simulink model "Bien1_simu"  (Simulink 9.1)
settings: Solver=VariableStepAuto  StartTime=0.0  StopTime=10.0  RelTol=1e-3
values from neighbouring files (symbols this model uses):
  m = [(m1*lc1^2)+m2*(l1^2+lc2^2+2*l1*lc2*cos(q2))+I1+I2 (m2*(lc2^2+l1*lc2*m2*cos(q2)+I2)) ... (first row only)    [brazomire.m]    (also in examvib3.m = 0.2533; fft estatica.m = [0:0.02:100]; fftestatica.m = [0:0.02:100])
  N = cat(1,N,b)    [ackerobs.m]    (also in espectograma.m = 128)
undefined symbols (not defined in the file or in its folder): As, Bs, CC, KK, uq, xq
libraries: mblibv1 x17
settings Model: LogicAnalyzerSignalOrdering=b2078105-ca7e-427e-be0d-a23da488db86  Creator=Dell  LastModifiedBy=Dell
settings DataIOCC: SaveFormat=Dataset
settings OptimizationCC: LifeSpan=auto
settings DebuggingCC: UnderspecifiedInitializationDetection=Simplified  MergeDetectMultiDrivingBlocksExec=error  SFUnexpectedBacktrackingDiag=error  SFNoUnconditionalDefaultTransitionDiag=error  SFExecutionAtInitializationDiag=warning
settings HardwareCC: ProdBitPerPointer=64  ProdBitPerSizeT=64  ProdBitPerPtrDiffT=64  ProdLargestAtomicFloat=Float  ProdIntDivRoundTo=Zero  ProdEndianess=LittleEndian  ProdWordSize=64  ProdHWDeviceType=Intel->x86-64 (Windows64)
settings ModelReferenceCC: PropagateSignalLabelsOutOfModel=on
settings GRTTargetCC: TargetLangStandard=C99 (ISO)  CombineOutputUpdateFcns=on  GRTInterface=off
settings ConfigComp: CovMetricSettings=dwe  CovHtmlReporting=off  CovSaveCumulativeToWorkspaceVar=off  CovSaveSingleToWorkspaceVar=off  CovExternalEMLEnable=on
settings SimscapeCC: SimscapeNormalizeSystem=off

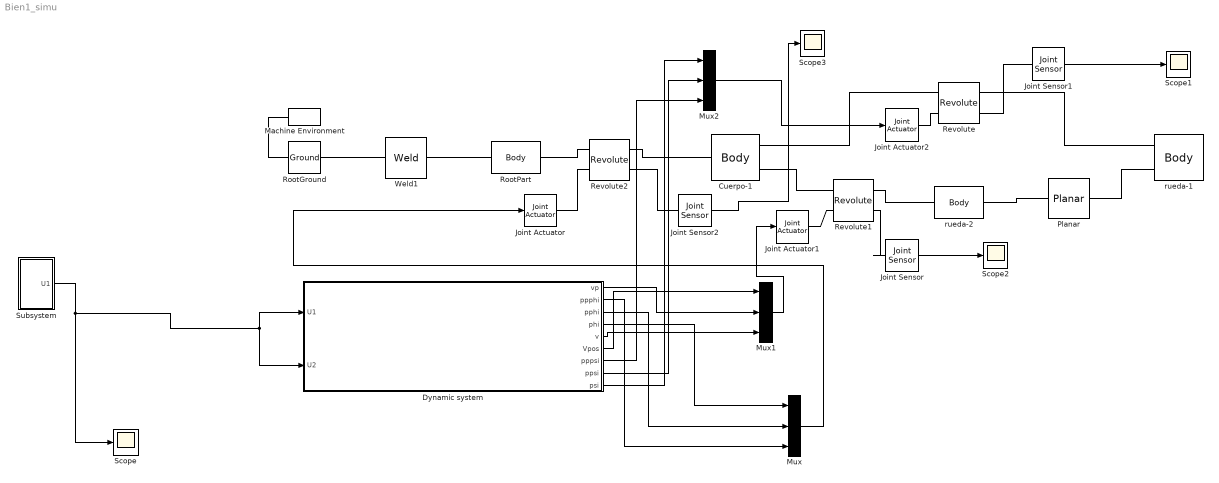
== system Bien1_simu ==
  Cuerpo-1 : mblibv1/Bodies/Body  LConnTagsString=CS2  RConnTagsString=CS3|CS4  UpdateFromCAD=on  DialogClass=MechanicalBodyBlock  Mass=0.199965  MassUnits=kg  InertiaUnits=kg*m^2  Inertia=[0.00141468,0,-1.2536e-08;0,0.00138764,6.39875e-09;-1.2536e-08,6.39875e-09,0.0027923]  Shape=Cylinder  ShapeDims=[1 1]  ShapeUnits=m  ShapeUse=false  Density=1  DensityUnits=kg/m^3  DensityUse=false  GraphicsMode=GFXFILE  GraphicsFileName=Segway - Cuerpo-1.STL  BodyColorSelMode=COLORPALETTE  BodyColor=[0.647059;0.619608;0.588235]  AttachedToCS=CS1  CG=Right$CG$[0.00341994 -0.0544159 8.19624e-07]$WORLD$WORLD$m$[1 0 0;0 1 0;0 0 1]$3x3 Transform$rad$WORLD$false$none  WorkingFrames=Right$CS1$[-0.18408 -0.111622 0]$WORLD$WORLD$m$[1 0 0;0 1 0;0 0 1]$3x3 Transform$rad$WORLD$false$none#Left$CS2$[0.00341994 -0.0544159 8.19624e-07]$WORLD$WORLD$m$[1 0 0;0 1 0;0 0 1]$3x3 Transform$rad$WORLD$true$none#Right$CS3$[0.19092 -0.111622 0]$WORLD$WORLD$m$[1 0 0;0 1 0;0 0 1]$3x3 Transform$rad$WORLD$true$none#Right$CS4$[0.19092 -0.111622 0]$WORLD$WORLD$m$[1 0 0;0 1 0;0 0 1]$3x3 Transform$rad$WORLD$true$none  CGPos=[0.00341994 -0.0544159 8.19624e-07]  CGRot=[1 0 0;0 1 0;0 0 1]  CS0Pos=[]  CS0Rot=[]  CS1Pos=[-0.18408 -0.111622 0]  CS1Rot=[1 0 0;0 1 0;0 0 1]  CS2Pos=[0.00341994 -0.0544159 8.19624e-07]  CS2Rot=[1 0 0;0 1 0;0 0 1]  CS3Pos=[0.19092 -0.111622 0]  CS3Rot=[1 0 0;0 1 0;0 0 1]  CS4Pos=[0.19092 -0.111622 0]  CS4Rot=[1 0 0;0 1 0;0 0 1]  CS5Pos=[]  CS5Rot=[]  CS6Pos=[]  CS6Rot=[]  CS7Pos=[]  CS7Rot=[]  CS8Pos=[]  CS8Rot=[]  CS9Pos=[]  CS9Rot=[]  CS10Pos=[]  CS10Rot=[]  CS11Pos=[]  CS11Rot=[]  CS12Pos=[]  CS12Rot=[]  CS13Pos=[]  CS13Rot=[]  CS14Pos=[]  CS14Rot=[]  CS15Pos=[]  CS15Rot=[]  CS16Pos=[]  CS16Rot=[]  CS17Pos=[]  CS17Rot=[]  CS18Pos=[]  CS18Rot=[]  CS19Pos=[]  CS19Rot=[]  CS20Pos=[]  CS20Rot=[]
      settings: SourceProductName=Simscape Multibody  SourceProductBaseCode=MS
  Dynamic system : Subsystem
  Joint Actuator : mblibv1/Sensors &  Actuators/Joint Actuator  UpdateFromCAD=off  PhysicalDomain=Mechanical  PortType=blob  ActuationStyle=Motion  AngleUnits=deg  ArcVelocityUnits=deg/s  ArcAccelerationUnits=deg/s^2  CoordPositionUnits=m  VelocityUnits=m/s  AccelerationUnits=m/s^2  ForceUnits=N  TorqueUnits=N*m  ActiveIO=on  Width=3  DialogClass=MechanicalActuatorBlock  Primitive=R1  ReferenceFrame=Absolute (World)
      settings: SourceProductName=Simscape Multibody  SourceProductBaseCode=MS
  Joint Actuator1 : mblibv1/Sensors &  Actuators/Joint Actuator  UpdateFromCAD=off  PhysicalDomain=Mechanical  PortType=blob  ActuationStyle=Motion  AngleUnits=deg  ArcVelocityUnits=rad/s  ArcAccelerationUnits=deg/s^2  CoordPositionUnits=m  VelocityUnits=m/s  AccelerationUnits=m/s^2  ForceUnits=N  TorqueUnits=N*m  ActiveIO=on  Width=3  DialogClass=MechanicalActuatorBlock  Primitive=R1  ReferenceFrame=Absolute (World)
      settings: SourceProductName=Simscape Multibody  SourceProductBaseCode=MS
  Joint Actuator2 : mblibv1/Sensors &  Actuators/Joint Actuator  UpdateFromCAD=off  PhysicalDomain=Mechanical  PortType=blob  ActuationStyle=Motion  AngleUnits=deg  ArcVelocityUnits=deg/s  ArcAccelerationUnits=deg/s^2  CoordPositionUnits=m  VelocityUnits=m/s  AccelerationUnits=m/s^2  ForceUnits=N  TorqueUnits=N*m  ActiveIO=on  Width=3  DialogClass=MechanicalActuatorBlock  Primitive=R1  ReferenceFrame=Absolute (World)
      settings: SourceProductName=Simscape Multibody  SourceProductBaseCode=MS
  Joint Sensor : mblibv1/Sensors &  Actuators/Joint Sensor  UpdateFromCAD=off  PhysicalDomain=Mechanical  PortType=blob  Muxed=on  Pose=off  Angle=on  AngleUnits=deg  ArcVelocity=off  ArcVelocityUnits=deg/s  ArcAcceleration=off  ArcAccelerationUnits=deg/s^2  CoordPosition=on  CoordPositionUnits=m  Velocity=off  VelocityUnits=m/s  Acceleration=off  AccelerationUnits=m/s^2  Quaternion=on  QuaternionDT=off  QuaternionDDT=off  QuaternionUnits=off  OutputVector=[1]  ActiveIO=on  Width=1  DialogClass=MechanicalSensorBlock  Primitive=R1  Force=off  ForceUnits=N  Torque=off  TorqueUnits=N-m  ReferenceFrame=Absolute (World)  ReactionSensedSide=Base  ReactionReferenceFrame=Absolute (World)  ReactionForce=off  ReactionForceUnits=N  ReactionMoment=off  ReactionMomentUnits=N-m
      settings: SourceProductName=Simscape Multibody  SourceProductBaseCode=MS
  Joint Sensor1 : mblibv1/Sensors &  Actuators/Joint Sensor  UpdateFromCAD=off  PhysicalDomain=Mechanical  PortType=blob  Muxed=on  Pose=off  Angle=on  AngleUnits=deg  ArcVelocity=off  ArcVelocityUnits=deg/s  ArcAcceleration=off  ArcAccelerationUnits=deg/s^2  CoordPosition=on  CoordPositionUnits=m  Velocity=off  VelocityUnits=m/s  Acceleration=off  AccelerationUnits=m/s^2  Quaternion=on  QuaternionDT=off  QuaternionDDT=off  QuaternionUnits=off  OutputVector=[1]  ActiveIO=on  Width=1  DialogClass=MechanicalSensorBlock  Primitive=R1  Force=off  ForceUnits=N  Torque=off  TorqueUnits=N-m  ReferenceFrame=Absolute (World)  ReactionSensedSide=Base  ReactionReferenceFrame=Absolute (World)  ReactionForce=off  ReactionForceUnits=N  ReactionMoment=off  ReactionMomentUnits=N-m
      settings: SourceProductName=Simscape Multibody  SourceProductBaseCode=MS
  Joint Sensor2 : mblibv1/Sensors &  Actuators/Joint Sensor  UpdateFromCAD=off  PhysicalDomain=Mechanical  PortType=blob  Muxed=on  Pose=off  Angle=on  AngleUnits=deg  ArcVelocity=off  ArcVelocityUnits=deg/s  ArcAcceleration=off  ArcAccelerationUnits=deg/s^2  CoordPosition=on  CoordPositionUnits=m  Velocity=off  VelocityUnits=m/s  Acceleration=off  AccelerationUnits=m/s^2  Quaternion=on  QuaternionDT=off  QuaternionDDT=off  QuaternionUnits=off  OutputVector=[1]  ActiveIO=on  Width=1  DialogClass=MechanicalSensorBlock  Primitive=R1  Force=off  ForceUnits=N  Torque=off  TorqueUnits=N-m  ReferenceFrame=Absolute (World)  ReactionSensedSide=Base  ReactionReferenceFrame=Absolute (World)  ReactionForce=off  ReactionForceUnits=N  ReactionMoment=off  ReactionMomentUnits=N-m
      settings: SourceProductName=Simscape Multibody  SourceProductBaseCode=MS
  Machine Environment : mblibv1/Bodies/Machine Environment  PortType=env  PhysicalDomain=Mechanical  DialogTemplateClass=MECH.MachineEnvironment  SyncWhenCopied=off  Gravity=[0 -9.81 0]  GravityUnits=m/s^2  GravityAsSignal=off  Dimensionality=Auto-detect  AnalysisType=Forward dynamics  LinearAssemblyTolerance=1e-3  LinearAssemblyToleranceUnits=m  AngularAssemblyTolerance=1e-3  AngularAssemblyToleranceUnits=rad  ConstraintSolverType=Stabilizing  ConstraintRelTolerance=1e-4  ConstraintAbsTolerance=1e-4  UseRobustSingularityHandling=off  RedundancyAnalysisToleranceType=Automatically select tolerance  RedundancyAnalysisTolerance=1e-14  StatePerturbationType=Fixed  PerturbationSize=1e-5  VisualizeMachine=on  BodyVisualizationType=Use model default body geometries  BodyColorSelMode=Use model default  DefaultBodyColor=[1 0 0]
      settings: SourceProductName=Simscape Multibody  SourceProductBaseCode=MS
  Mux : Mux  Inputs=3
  Mux1 : Mux  Inputs=3
  Mux2 : Mux  Inputs=3
  Planar : mblibv1/Joints/Planar  LConnTagsString=__newl0  RConnTagsString=__newr0  UpdateFromCAD=on  NumSAPorts=0  CutJoint=off  MarkAsCut=off  Primitives=prismatic_prismatic  PrimitiveProps=P1$WORLD$[0,1,0]$prismatic#P2$WORLD$[0,0,1]$prismatic#R1$WORLD$[-1,0,0]$revolute  DialogClass=JointBlock  P1Axis=[0,1,0]  P2Axis=[0,0,1]  R1Axis=[-1,0,0]
      settings: SourceProductName=Simscape Multibody  SourceProductBaseCode=MS
  Revolute : mblibv1/Joints/Revolute  LConnTagsString=__newl0|SA1  RConnTagsString=__newr0|SA1  UpdateFromCAD=on  NumSAPorts=2  CutJoint=off  MarkAsCut=off  Primitives=prismatic  PrimitiveProps=R1$World$[-1,0,0]$revolute  DialogClass=JointBlock  R1Axis=[-1,0,0]
      settings: SourceProductName=Simscape Multibody  SourceProductBaseCode=MS
  Revolute1 : mblibv1/Joints/Revolute  LConnTagsString=__newl0|SA1  RConnTagsString=__newr0|SA1  UpdateFromCAD=on  NumSAPorts=2  CutJoint=off  MarkAsCut=off  Primitives=prismatic  PrimitiveProps=R1$World$[-1,0,0]$revolute  DialogClass=JointBlock  R1Axis=[-1,0,0]
      settings: SourceProductName=Simscape Multibody  SourceProductBaseCode=MS
  Revolute2 : mblibv1/Joints/Revolute  LConnTagsString=__newl0|SA1  RConnTagsString=__newr0|SA1  UpdateFromCAD=on  NumSAPorts=2  CutJoint=off  MarkAsCut=off  Primitives=prismatic  PrimitiveProps=R1$World$[-1,0,0]$revolute  DialogClass=JointBlock  R1Axis=[-1,0,0]
      settings: SourceProductName=Simscape Multibody  SourceProductBaseCode=MS
  RootGround : mblibv1/Bodies/Ground  UpdateFromCAD=on  LeftPortType=env  RightPortType=workingframe  PhysicalDomain=Mechanical  DialogClass=GroundBlock  CoordPosition=[0.00341994,-0.0977707,1.98458e-07]  CoordPositionUnits=m  StateVectorMgrId=0  MachineId=[1 0]  ShowEnvPort=on  ParameterChecksum=[377609271, 2150916510, 2923505872, 3171247844]  TopologyChecksum=[4158908636, 1793340263, 2655611642, 3121996530]
      settings: SourceProductName=Simscape Multibody  SourceProductBaseCode=MS
  RootPart : mblibv1/Bodies/Body  LConnTagsString=CS3  RConnTagsString=CS2  UpdateFromCAD=on  DialogClass=MechanicalBodyBlock  Mass=0  MassUnits=kg  InertiaUnits=kg*m^2  Inertia=[0,0,0;0,0,0;0,0,0]  Shape=Cylinder  ShapeDims=[1 1]  ShapeUnits=m  ShapeUse=false  Density=1  DensityUnits=kg/m^3  DensityUse=false  GraphicsMode=MACHINE_DEFAULT  BodyColorSelMode=MACHINE_DEFAULT  BodyColor=[1;0;0]  AttachedToCS=CS1  CG=Right$CG$[0.00341994 -0.0977707 1.98458e-07]$WORLD$WORLD$m$[1 0 0;0 1 0;0 0 1]$3x3 Transform$rad$WORLD$false$none  WorkingFrames=Right$CS1$[0 0 0]$WORLD$WORLD$m$[1 0 0;0 1 0;0 0 1]$3x3 Transform$rad$WORLD$false$none#Right$CS2$[0.00341994 -0.0544159 8.19624e-07]$WORLD$WORLD$m$[1 0 0;0 1 0;0 0 1]$3x3 Transform$rad$WORLD$true$none#Left$CS3$[0.00341994 -0.0977707 1.98458e-07]$WORLD$WORLD$m$[1 0 0;0 1 0;0 0 1]$3x3 Transform$rad$WORLD$true$none  CGPos=[0.00341994 -0.0977707 1.98458e-07]  CGRot=[1 0 0;0 1 0;0 0 1]  CS0Pos=[]  CS0Rot=[]  CS1Pos=[0 0 0]  CS1Rot=[1 0 0;0 1 0;0 0 1]  CS2Pos=[0.00341994 -0.0544159 8.19624e-07]  CS2Rot=[1 0 0;0 1 0;0 0 1]  CS3Pos=[0.00341994 -0.0977707 1.98458e-07]  CS3Rot=[1 0 0;0 1 0;0 0 1]  CS4Pos=[]  CS4Rot=[]  CS5Pos=[]  CS5Rot=[]  CS6Pos=[]  CS6Rot=[]  CS7Pos=[]  CS7Rot=[]  CS8Pos=[]  CS8Rot=[]  CS9Pos=[]  CS9Rot=[]  CS10Pos=[]  CS10Rot=[]  CS11Pos=[]  CS11Rot=[]  CS12Pos=[]  CS12Rot=[]  CS13Pos=[]  CS13Rot=[]  CS14Pos=[]  CS14Rot=[]  CS15Pos=[]  CS15Rot=[]  CS16Pos=[]  CS16Rot=[]  CS17Pos=[]  CS17Rot=[]  CS18Pos=[]  CS18Rot=[]  CS19Pos=[]  CS19Rot=[]  CS20Pos=[]  CS20Rot=[]
      settings: SourceProductName=Simscape Multibody  SourceProductBaseCode=MS
  Scope{,1..3} (4 alike) : Scope
  Subsystem : Subsystem
  Weld1 : mblibv1/Joints/Weld  LConnTagsString=__newl0  RConnTagsString=__newr0  UpdateFromCAD=on  NumSAPorts=0  CutJoint=off  MarkAsCut=off  Primitives=weld  PrimitiveProps=W$WORLD$[0.57735,0.57735,0.57735]$weld  DialogClass=JointBlock  WAxis=[0.57735,0.57735,0.57735]
      settings: SourceProductName=Simscape Multibody  SourceProductBaseCode=MS
  rueda-1 : mblibv1/Bodies/Body  LConnTagsString=CS2|CS3  UpdateFromCAD=on  DialogClass=MechanicalBodyBlock  Mass=0.312941  MassUnits=kg  InertiaUnits=kg*m^2  Inertia=[0.000332401,0,0;0,0.000332401,0;0,0,0.000634107]  Shape=Cylinder  ShapeDims=[1 1]  ShapeUnits=m  ShapeUse=false  Density=1  DensityUnits=kg/m^3  DensityUse=false  GraphicsMode=GFXFILE  GraphicsFileName=Segway - rueda-1.STL  BodyColorSelMode=COLORPALETTE  BodyColor=[1;1;1]  AttachedToCS=CS1  CG=Right$CG$[-0.17158 -0.111622 0]$WORLD$WORLD$m$[0 0 -1;0 1 0;1 0 0]$3x3 Transform$rad$WORLD$false$none  WorkingFrames=Right$CS1$[-0.15908 -0.111622 0]$WORLD$WORLD$m$[0 0 -1;0 1 0;1 0 0]$3x3 Transform$rad$WORLD$false$none#Left$CS2$[0.19092 -0.111622 0]$WORLD$WORLD$m$[1 0 0;0 1 0;0 0 1]$3x3 Transform$rad$WORLD$true$none#Left$CS3$[0.16592 -0.111622 0]$WORLD$WORLD$m$[1 0 0;0 1 0;0 0 1]$3x3 Transform$rad$WORLD$true$none  CGPos=[-0.17158 -0.111622 0]  CGRot=[0 0 -1;0 1 0;1 0 0]  CS0Pos=[]  CS0Rot=[]  CS1Pos=[-0.15908 -0.111622 0]  CS1Rot=[0 0 -1;0 1 0;1 0 0]  CS2Pos=[0.19092 -0.111622 0]  CS2Rot=[1 0 0;0 1 0;0 0 1]  CS3Pos=[0.16592 -0.111622 0]  CS3Rot=[1 0 0;0 1 0;0 0 1]  CS4Pos=[]  CS4Rot=[]  CS5Pos=[]  CS5Rot=[]  CS6Pos=[]  CS6Rot=[]  CS7Pos=[]  CS7Rot=[]  CS8Pos=[]  CS8Rot=[]  CS9Pos=[]  CS9Rot=[]  CS10Pos=[]  CS10Rot=[]  CS11Pos=[]  CS11Rot=[]  CS12Pos=[]  CS12Rot=[]  CS13Pos=[]  CS13Rot=[]  CS14Pos=[]  CS14Rot=[]  CS15Pos=[]  CS15Rot=[]  CS16Pos=[]  CS16Rot=[]  CS17Pos=[]  CS17Rot=[]  CS18Pos=[]  CS18Rot=[]  CS19Pos=[]  CS19Rot=[]  CS20Pos=[]  CS20Rot=[]
      settings: SourceProductName=Simscape Multibody  SourceProductBaseCode=MS
  rueda-2 : mblibv1/Bodies/Body  LConnTagsString=CS3  RConnTagsString=CS2  UpdateFromCAD=on  DialogClass=MechanicalBodyBlock  Mass=0.312941  MassUnits=kg  InertiaUnits=kg*m^2  Inertia=[0.000332401,0,0;0,0.000332401,0;0,0,0.000634107]  Shape=Cylinder  ShapeDims=[1 1]  ShapeUnits=m  ShapeUse=false  Density=1  DensityUnits=kg/m^3  DensityUse=false  GraphicsMode=GFXFILE  GraphicsFileName=Segway - rueda-2.STL  BodyColorSelMode=COLORPALETTE  BodyColor=[1;1;1]  AttachedToCS=CS1  CG=Right$CG$[0.17842 -0.111622 0]$WORLD$WORLD$m$[0 0 -1;-0.309052 0.951045 0;0.951045 0.309052 0]$3x3 Transform$rad$WORLD$false$none  WorkingFrames=Right$CS1$[0.19092 -0.111622 0]$WORLD$WORLD$m$[0 0 -1;-0.309052 0.951045 0;0.951045 0.309052 0]$3x3 Transform$rad$WORLD$false$none#Right$CS2$[0.16592 -0.111622 0]$WORLD$WORLD$m$[1 0 0;0 1 0;0 0 1]$3x3 Transform$rad$WORLD$true$none#Left$CS3$[0.19092 -0.111622 0]$WORLD$WORLD$m$[1 0 0;0 1 0;0 0 1]$3x3 Transform$rad$WORLD$true$none  CGPos=[0.17842 -0.111622 0]  CGRot=[0 0 -1;-0.309052 0.951045 0;0.951045 0.309052 0]  CS0Pos=[]  CS0Rot=[]  CS1Pos=[0.19092 -0.111622 0]  CS1Rot=[0 0 -1;-0.309052 0.951045 0;0.951045 0.309052 0]  CS2Pos=[0.16592 -0.111622 0]  CS2Rot=[1 0 0;0 1 0;0 0 1]  CS3Pos=[0.19092 -0.111622 0]  CS3Rot=[1 0 0;0 1 0;0 0 1]  CS4Pos=[]  CS4Rot=[]  CS5Pos=[]  CS5Rot=[]  CS6Pos=[]  CS6Rot=[]  CS7Pos=[]  CS7Rot=[]  CS8Pos=[]  CS8Rot=[]  CS9Pos=[]  CS9Rot=[]  CS10Pos=[]  CS10Rot=[]  CS11Pos=[]  CS11Rot=[]  CS12Pos=[]  CS12Rot=[]  CS13Pos=[]  CS13Rot=[]  CS14Pos=[]  CS14Rot=[]  CS15Pos=[]  CS15Rot=[]  CS16Pos=[]  CS16Rot=[]  CS17Pos=[]  CS17Rot=[]  CS18Pos=[]  CS18Rot=[]  CS19Pos=[]  CS19Rot=[]  CS20Pos=[]  CS20Rot=[]
      settings: SourceProductName=Simscape Multibody  SourceProductBaseCode=MS
  wires:
  Joint Sensor2/1 -> Scope3/1
  Mux2/1 -> Joint Actuator2/1
  Joint Sensor/1 -> Scope2/1
  Joint Sensor1/1 -> Scope1/1
  Subsystem/1("U1 ") -> Scope/1, Dynamic system/1(U1), Dynamic system/2(U2)
  Mux/1 -> Joint Actuator/1
  Dynamic system/4(phi) -> Mux/1
  Dynamic system/3(pphi) -> Mux/2
  Dynamic system/2(ppphi) -> Mux/3
  Dynamic system/9(psi) -> Mux2/1
  Dynamic system/8(ppsi) -> Mux2/2
  Dynamic system/7(pppsi) -> Mux2/3
  Dynamic system/6(Vpos) -> Mux1/1
  Dynamic system/5(v) -> Mux1/3
  Dynamic system/1(vp) -> Mux1/2
  Mux1/1 -> Joint Actuator1/1
  connections:
  Joint Sensor2/LConn1 -- Revolute2/RConn2
  Joint Sensor1/LConn1 -- Revolute/RConn2
  Joint Sensor/LConn1 -- Revolute1/RConn2
  Revolute2/LConn2 -- Joint Actuator/RConn1
  Joint Actuator2/RConn1 -- Revolute/LConn2
  RootGround/LConn1 -- Machine Environment/RConn1
  Weld1/RConn1 -- RootPart/LConn1
  Revolute1/RConn1 -- rueda-2/LConn1
  RootGround/RConn1 -- Weld1/LConn1
  Revolute1/LConn1 -- Cuerpo-1/RConn2
  Revolute/RConn1 -- rueda-1/LConn1
  Planar/RConn1 -- rueda-1/LConn2
  Cuerpo-1/RConn1 -- Revolute/LConn1
  Revolute2/RConn1 -- Cuerpo-1/LConn1
  Revolute2/LConn1 -- RootPart/RConn1
  rueda-2/RConn1 -- Planar/LConn1
  Joint Actuator1/RConn1 -- Revolute1/LConn2

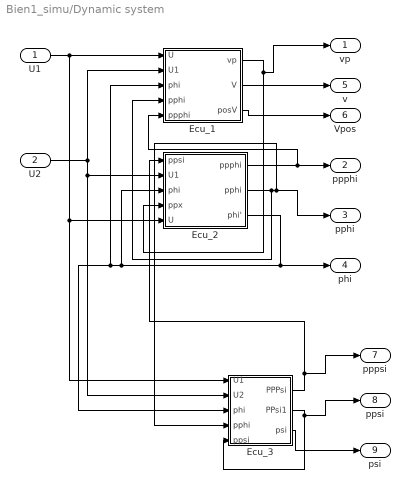
== system Bien1_simu/Dynamic system ==
  U1 : Inport
  U2 : Inport  Port=2
  Ecu_1 : Subsystem
  Ecu_2 : Subsystem
  Ecu_3 : Subsystem
  vp : Outport
  ppphi : Outport  Port=2
  pphi : Outport  Port=3
  phi : Outport  Port=4
  v : Outport  Port=5
  Vpos : Outport  Port=6
  pppsi : Outport  Port=7
  ppsi : Outport  Port=8
  psi : Outport  Port=9
  wires:
  Ecu_1/3(posV) -> Vpos/1
  Ecu_1/2(V) -> v/1
  Ecu_1/1(vp) -> Ecu_2/4(" ppx"), vp/1
  U1/1 -> Ecu_1/1(U), Ecu_2/5(" U"), Ecu_3/1(U1)
  U2/1 -> Ecu_1/2(U1), Ecu_2/2(U1), Ecu_3/2(U2)
  Ecu_2/1(ppphi) -> Ecu_1/5(ppphi), ppphi/1
  Ecu_2/2(pphi) -> Ecu_1/4(pphi), Ecu_3/4(pphi), pphi/1
  Ecu_2/3(phi') -> Ecu_1/3(phi), Ecu_3/3(phi), Ecu_2/3(phi), phi/1
  Ecu_3/2(PPsi1) -> ppsi/1, Ecu_3/5(ppsi)
  Ecu_3/1(PPPsi) -> pppsi/1, Ecu_2/1(" ppsi")
  Ecu_3/3(psi) -> psi/1

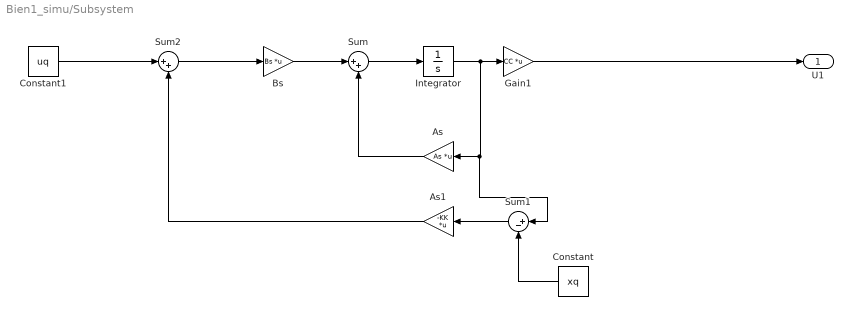
== system Bien1_simu/Subsystem ==
  As : Gain  Gain=As  Multiplication=Matrix(K*u)
  As1 : Gain  Gain=-KK  Multiplication=Matrix(K*u)
  Bs : Gain  Gain=Bs  Multiplication=Matrix(K*u)
  Constant : Constant  Value=xq
  Constant1 : Constant  Value=uq
  Gain1 : Gain  Gain=CC  Multiplication=Matrix(K*u)
  Integrator : Integrator  InitialCondition=[2;0;10;0]
  Sum : Sum  Inputs=|++
  Sum1 : Sum  Inputs=|+-
  Sum2 : Sum  Inputs=|++
  "U1 " : Outport
  wires:
  As1/1 -> Sum2/2
  Sum1/1 -> As1/1
  Constant/1 -> Sum1/2
  Integrator/1 -> Gain1/1, As/1, Sum1/1
  Constant1/1 -> Sum2/1
  Sum2/1 -> Bs/1
  As/1 -> Sum/2
  Gain1/1 -> "U1 "/1
  Bs/1 -> Sum/1
  Sum/1 -> Integrator/1

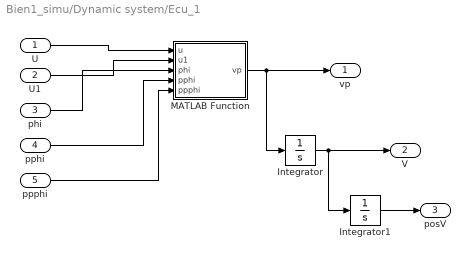
== system Bien1_simu/Dynamic system/Ecu_1 ==
  U : Inport
  U1 : Inport  Port=2
  phi : Inport  Port=3
  pphi : Inport  Port=4
  ppphi : Inport  Port=5
  Integrator : Integrator
  Integrator1 : Integrator
  MATLAB Function : MATLAB Function  TreatAsAtomicUnit=on
  vp : Outport
  V : Outport  Port=2
  posV : Outport  Port=3
  wires:
  MATLAB Function/1(vp) -> Integrator/1, vp/1
  U/1 -> MATLAB Function/1(u)
  U1/1 -> MATLAB Function/2(u1)
  phi/1 -> MATLAB Function/3(phi)
  pphi/1 -> MATLAB Function/4(pphi)
  ppphi/1 -> MATLAB Function/5(ppphi)
  Integrator/1 -> Integrator1/1, V/1
  Integrator1/1 -> posV/1

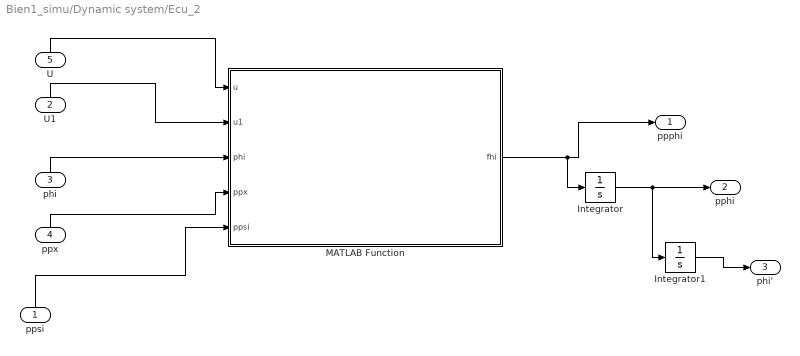
== system Bien1_simu/Dynamic system/Ecu_2 ==
  " ppsi" : Inport
  U1 : Inport  Port=2
  phi : Inport  Port=3
  " ppx" : Inport  Port=4
  " U" : Inport  Port=5
  Integrator : Integrator
  Integrator1 : Integrator
  MATLAB Function : MATLAB Function  TreatAsAtomicUnit=on
  ppphi : Outport
  pphi : Outport  Port=2
  phi' : Outport  Port=3
  wires:
  " U"/1 -> MATLAB Function/1(u)
  U1/1 -> MATLAB Function/2(u1)
  phi/1 -> MATLAB Function/3(phi)
  " ppx"/1 -> MATLAB Function/4(ppx)
  " ppsi"/1 -> MATLAB Function/5(ppsi)
  MATLAB Function/1(fhi) -> Integrator/1, ppphi/1
  Integrator/1 -> Integrator1/1, pphi/1
  Integrator1/1 -> phi'/1

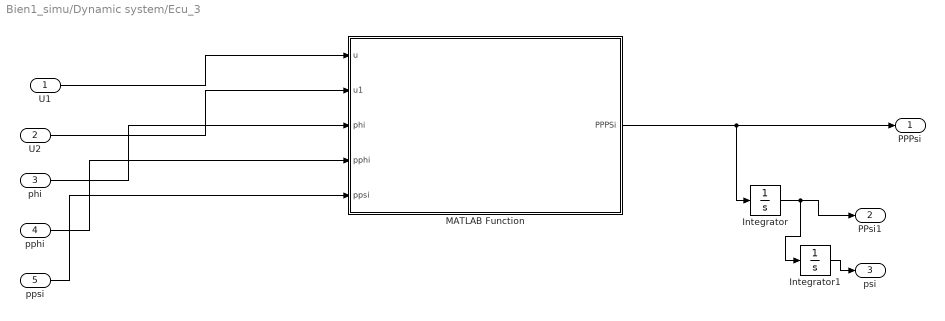
== system Bien1_simu/Dynamic system/Ecu_3 ==
  U1 : Inport
  U2 : Inport  Port=2
  phi : Inport  Port=3
  pphi : Inport  Port=4
  ppsi : Inport  Port=5
  Integrator : Integrator
  Integrator1 : Integrator
  MATLAB Function : MATLAB Function  TreatAsAtomicUnit=on
  PPPsi : Outport
  PPsi1 : Outport  Port=2
  psi : Outport  Port=3
  wires:
  U2/1 -> MATLAB Function/2(u1)
  U1/1 -> MATLAB Function/1(u)
  MATLAB Function/1(PPPSi) -> Integrator/1, PPPsi/1
  Integrator/1 -> Integrator1/1, PPsi1/1
  Integrator1/1 -> psi/1
  phi/1 -> MATLAB Function/3(phi)
  pphi/1 -> MATLAB Function/4(pphi)
  ppsi/1 -> MATLAB Function/5(ppsi)

== matlab function Dynamic system/Ecu_2/MATLAB Function ==
  data: u input double; fhi output double; u1 input double; phi input double; ppx input double; ppsi input double
function fhi = fcn(u,u1,phi,ppx,ppsi)
%#codegen
mb=13.30
d=.1300

chi=mb*d*d+I1;

ppphi= (-(u1+u2)-(mb*d*cos(phi)*ppx)+(mb*d*d*I1+I2)*sin(phi)*cos(phi)*ppsi*ppsi+mb*g*d*sin(phi))/chi;

== matlab function Dynamic system/Ecu_1/MATLAB Function ==
  data: u input double; vp output double; u1 input double; phi input double; pphi input double; ppphi input double
function vp = fcn(u,u1,phi,pphi,ppphi)
%#codegen

Rho=mb*(2*mw+(2*I1/R));

y = ((u1/R+u/R)-(mb*d*cos(phi)*ppphi)+(mb1*d*sin(phi)*phi*phi))/Rho;

== matlab function Dynamic system/Ecu_3/MATLAB Function ==
  data: u input double; PPPSi output double; u1 input double; phi input double; pphi input double; ppsi input double
function PPPSi = fcn(u,u1,phi,pphi,ppsi)
%#codegen

theta=2*((mw+I1/R)*L^2)+I2*sin(phi)*sin(phi)+I3*cos(phi)*cos(phi)+m2*d*d*sin(phi)

pppsi= ((L/R)*(u-u1)-2*(mb*d*d+I2-I3)*sin(phi)*cos(phi)*ppsi*pphi)/theta;
